simulink model "Test_Model_HR12_2016"  (R2016b)
settings: Solver=FixedStepAuto  StartTime=0.0  StopTime=length(ipoint)  FixedStep=dt  RelTol=1e-3
values from neighbouring files (symbols this model uses):
  Cbx_cyl_fill_efy_intk_mfld_prs_atm_prs_cor_cho = true    [Calib_mdl_RSA.m]
  Cbx_cyl_fill_efy_opt_cho = false    [Calib_mdl_RSA.m]
  Cbx_cyl_fill_igr_opt_cho = false    [Calib_mdl_RSA.m]
  Cbx_ex_vvt_conf = true    [Calib_mdl_RSA.m]
  Cnx_cyl_fill_ex_mfld_prs_cor_cho = 0    [Cal_basic.m]
  Cnx_cyl_nr_conf = 3    [Cal_basic.m]
  Cxx_cyl_fill_efy_drv_max = 20    [Calib_mdl_RSA.m]
  Cxx_cyl_fill_efy_dyn_max = 0.15    [Calib_mdl_RSA.m]
  Cxx_cyl_fill_efy_dyn_min = 0    [Calib_mdl_RSA.m]
  Cxx_cyl_fill_efy_dz = 0.45    [Calib_mdl_RSA.m]
  Cxx_cyl_fill_efy_ovlp_angl = 66    [Calib_mdl_RSA.m]
  Cxx_cyl_fill_efy_vvt_ofs = 0    [Calib_mdl_RSA.m]
  Cxx_cyl_fill_trap_area_h_thd = 0.2    [Cal_basic.m]
  Cxx_cyl_fill_trap_area_l_thd = 0.1    [Cal_basic.m]
  Cxx_cyl_fill_trap_efy_dz_l_thd = 1    [Cal_basic.m]
  Cxx_cyl_fill_trap_efy_dz_neg_slop = -0.5    [Cal_basic.m]
  Cxx_cyl_fill_trap_efy_dz_pos_slop = 0.5    [Cal_basic.m]
  Cxx_cyl_fill_trap_vvt_ovlp_angl = 120    [Calib_mdl_RSA.m]
  Cxx_cyl_vol = 3.9961e-04*3    (= 0.00119883)    [Cal_basic.m]    (also in Calib_mdl_RSA.m = 0.00119900004938)
  Cxx_min_cyl_fill_mdl_ex_mfld_prs_rat_cor = 0    [Cal_basic.m]
  Nnx_eng_run_stt = 2    [Calib_mdl_RSA.m]
  Nxx_atm_kpa = 101.3    [Cal_basic.m]
  Nxx_k_degc = 273.15    [Cal_basic.m]
  Nxx_kilo_bas = 1000    [Cal_basic.m]
  Nxx_wht_pgc_j_kg = 287    [Cal_basic.m]
undefined symbols (not defined in the file or in its folder): Cxx_egr_spc_heat, Cxx_thr_spc_heat, docblock, MapFilling_Aspirated
libraries: AEMS_Standard_Library x78, simulink x2
(part 1 of 5)
settings Model: Creator=a002701  LastModifiedBy=a002701

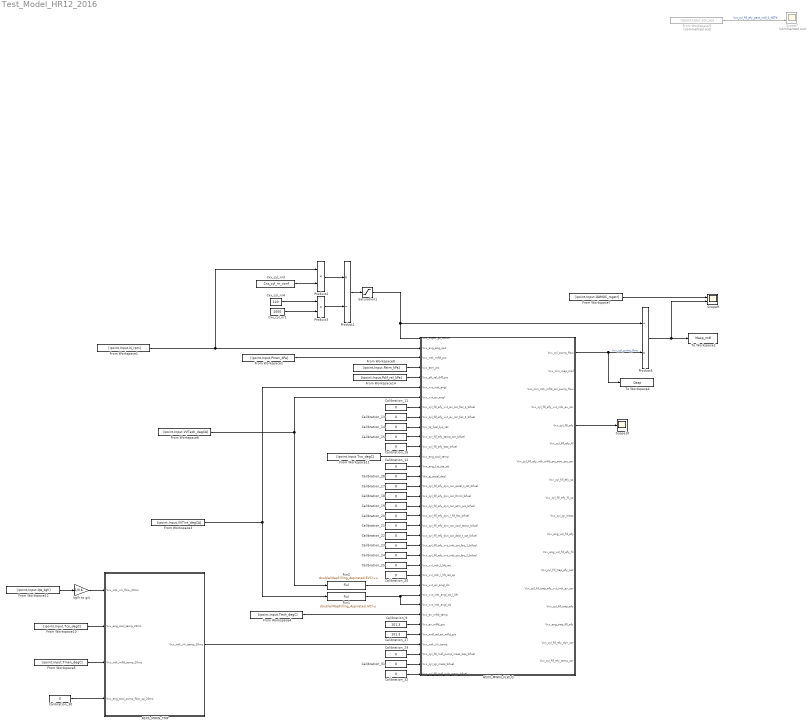
== system Test_Model_HR12_2016 ==
  ASXX_MWIN_FLW_G : Subsystem
  ASXX_MWIN_TMP : Subsystem  Tag=[MODULE]
  Calibration_{11..26,28..32} (21 alike) : Constant  Value=0  OutDataTypeStr=Inherit: Inherit via back propagation
  Calibration_27 : Constant  Value=101.3  OutDataTypeStr=Inherit: Inherit via back propagation
  Calibration_9 : Constant  Value=101.3  OutDataTypeStr=Inherit: Inherit via back propagation
  Cxx_cyl_nr1 : Constant  Value=1000  OutDataTypeStr=single
  Cxx_cyl_nr3 : Constant  Value=Cnx_cyl_nr_conf
  Cxx_cyl_nr4 : Constant  Value=120  OutDataTypeStr=single
  Fcn1 : Fcn  Expr=double(MapFilling_Aspirated.IVC)-u
  Fcn2 : Fcn  Expr=double(MapFilling_Aspirated.EVC)+u
  From Workspace1 : FromWorkspace  VariableName=[ipoint,Input.N_rpm]  SampleTime=0  Interpolate=off  OutputAfterFinalValue=Holding final value
  From Workspace10 : FromWorkspace  VariableName=[ipoint,Input.Tco_degC]  SampleTime=1  Interpolate=off  OutputAfterFinalValue=Holding final value
  From Workspace11 : FromWorkspace  VariableName=[ipoint,Input.Tco_degC]  SampleTime=1  Interpolate=off  OutputAfterFinalValue=Holding final value
  From Workspace12 : FromWorkspace  VariableName=[ipoint,Input.QA_kgh]  SampleTime=1  Interpolate=off  OutputAfterFinalValue=Holding final value
  From Workspace14 : FromWorkspace  VariableName=[ipoint,Input.Pdif_rel_kPa]  SampleTime=1  Interpolate=off  OutputAfterFinalValue=Holding final value
  From Workspace2 : FromWorkspace  VariableName=[ipoint,Input.Pman_kPa]  SampleTime=0  Interpolate=off  OutputAfterFinalValue=Holding final value
  From Workspace3 : FromWorkspace  VariableName=[ipoint,Input.VVTint_degCA]  SampleTime=0  Interpolate=off  OutputAfterFinalValue=Holding final value
  From Workspace4 : FromWorkspace  VariableName=[ipoint,Input.Texh_degC]  SampleTime=0  Interpolate=off  OutputAfterFinalValue=Holding final value
  From Workspace5 : FromWorkspace  VariableName=[ipoint,Input.Tman_degC]  SampleTime=0  Interpolate=off  OutputAfterFinalValue=Holding final value
  From Workspace6 : FromWorkspace  VariableName=[ipoint,Input.VVTexh_degCA]  SampleTime=0  Interpolate=off  OutputAfterFinalValue=Holding final value
  From Workspace7 : FromWorkspace  VariableName=[ipoint,Input.QAMGC_mgstr]  SampleTime=1  Interpolate=off  OutputAfterFinalValue=Holding final value
  From Workspace8 : FromWorkspace  VariableName=[ipoint,Input.Patm_kPa]  SampleTime=1  Interpolate=off  OutputAfterFinalValue=Holding final value
  From Workspace9 : FromWorkspace  Commented=on  VariableName=[ipoint,Input.eta_wu]  SampleTime=1  Interpolate=off  OutputAfterFinalValue=Holding final value
  Product1 : Product  Inputs=*/  OutDataTypeStr=Inherit: Inherit via back propagation
  Product2 : Product  Inputs=**  OutDataTypeStr=Inherit: Inherit via back propagation
  Product3 : Product  Inputs=**  OutDataTypeStr=Inherit: Inherit via back propagation
  Product5 : Product  Inputs=/*  OutDataTypeStr=Inherit: Inherit via back propagation
  Saturation1 : Saturate  UpperLimit=1  LowerLimit=0
      settings: AttributesFormatString=<limits=%<UpperLimit>/%<LowerLimit>>
  Scope10 : Scope
  Scope7 : Scope  Commented=on  NumInputPorts=2
  Scope9 : Scope  NumInputPorts=2
  To Workspace2 : ToWorkspace  VariableName=Masp_mdl  SampleTime=1
  To Workspace4 : ToWorkspace  VariableName=Qasp  SampleTime=1
  kg/h to g/s : Gain  Gain=1/3.6
  wires:
  From Workspace3/1 -> Fcn1/1, ASXX_MWIN_FLW_G/6(Vxx_vvt_intk_angl)
  From Workspace6/1 -> Fcn2/1, ASXX_MWIN_FLW_G/7(Vxx_vvt_ex_angl)
  ASXX_MWIN_TMP/1(Vxx_intk_vlv_temp_20ms) -> ASXX_MWIN_FLW_G/32(Vxx_intk_vlv_temp)
  From Workspace2/1 -> ASXX_MWIN_FLW_G/3(Vxx_intk_mfld_prs)
  From Workspace4/1 -> ASXX_MWIN_FLW_G/29(Vxx_ex_mfld_temp)
  Fcn1/1 -> ASXX_MWIN_FLW_G/27(Vxx_vvt_intk_angl_cls_l_lift), ASXX_MWIN_FLW_G/28(Vxx_vvt_intk_angl_cls)
  Fcn2/1 -> ASXX_MWIN_FLW_G/26(Vxx_vvt_ex_angl_cls)
  From Workspace7/1 -> Scope9/1
  Product2/1 -> Product1/1
  Product1/1 -> Saturation1/1
  Product3/1 -> Product1/2
  From Workspace1/1 -> Product2/1, ASXX_MWIN_FLW_G/2(Vxx_avg_eng_spd)
  Cxx_cyl_nr4/1 -> Product3/1
  Cxx_cyl_nr1/1 -> Product3/2
  Cxx_cyl_nr3/1 -> Product2/2
  Saturation1/1 -> ASXX_MWIN_FLW_G/1(Vxx_mgstr_gs_convs), Product5/1
  From Workspace9/1 -> Scope7/2  "Vxt_cyl_fill_efy_para_mdl_0_XETK"
  From Workspace14/1 -> ASXX_MWIN_FLW_G/5(Vxx_pft_rel_diff_prs)
  Calibration_11/1 -> ASXX_MWIN_FLW_G/8(Vxx_cyl_fill_efy_vvt_ex_cor_fac_1_bifuel)
  Calibration_13/1 -> ASXX_MWIN_FLW_G/9(Vxx_cyl_fill_efy_vvt_ex_cor_fac_2_bifuel)
  Calibration_14/1 -> ASXX_MWIN_FLW_G/10(Vxx_tq_fuel_typ_rat)
  Calibration_15/1 -> ASXX_MWIN_FLW_G/11(Vxx_cyl_fill_efy_temp_cor_bifuel)
  Calibration_16/1 -> ASXX_MWIN_FLW_G/12(Vxx_cyl_fill_efy_bas_bifuel)
  Calibration_17/1 -> ASXX_MWIN_FLW_G/16(Vxx_cyl_fill_efy_dyn_cor_accel_t_cst_bifuel)
  Calibration_18/1 -> ASXX_MWIN_FLW_G/17(Vxx_cyl_fill_efy_dyn_cor_thrml_bifuel)
  Calibration_19/1 -> ASXX_MWIN_FLW_G/18(Vxx_cyl_fill_efy_dyn_cor_atm_prs_bifuel)
  Calibration_20/1 -> ASXX_MWIN_FLW_G/19(Vxx_cyl_fill_efy_dyn_l_fill_fac_bifuel)
  Calibration_21/1 -> ASXX_MWIN_FLW_G/20(Vxx_cyl_fill_efy_dyn_cor_cool_temp_bifuel)
  Calibration_22/1 -> ASXX_MWIN_FLW_G/21(Vxx_cyl_fill_efy_dyn_cor_decl_t_cst_bifuel)
  Calibration_23/1 -> ASXX_MWIN_FLW_G/22(Vxx_cyl_fill_efy_vvt_intk_cor_fac_1_bifuel)
  Calibration_24/1 -> ASXX_MWIN_FLW_G/23(Vxx_cyl_fill_efy_vvt_intk_cor_fac_2_bifuel)
  Calibration_25/1 -> ASXX_MWIN_FLW_G/24(Vxx_vvl_intk_l_lift_rat)
  Calibration_26/1 -> ASXX_MWIN_FLW_G/25(Vxx_vvl_intk_l_lift_rat_sp)
  Calibration_27/1 -> ASXX_MWIN_FLW_G/31(Vxx_mdl_ref_ex_mfld_prs)
  Calibration_12/1 -> ASXX_MWIN_FLW_G/14(Vnx_eng_1st_sta_stt)
  Calibration_28/1 -> ASXX_MWIN_FLW_G/15(Vbx_aj_accel_decl)
  From Workspace8/1 -> ASXX_MWIN_FLW_G/4(Vxx_atm_prs)
  Calibration_9/1 -> ASXX_MWIN_FLW_G/30(Vxx_ex_mfld_prs)
  From Workspace11/1 -> ASXX_MWIN_FLW_G/13(Vxx_eng_cool_temp)
  ASXX_MWIN_FLW_G/1(Vxx_cyl_pump_flow) -> To Workspace4/1, Product5/2  "Vxx_cyl_pump_flow"
  Product5/1 -> Scope9/2, To Workspace2/1
  ASXX_MWIN_FLW_G/5(Vxx_cyl_fill_efy) -> Scope10/1
  Calibration_30/1 -> ASXX_MWIN_TMP/4(Vxx_eng_cool_pump_flow_sp_20ms)
  From Workspace10/1 -> ASXX_MWIN_TMP/2(Vxx_eng_cool_temp_20ms)
  From Workspace5/1 -> ASXX_MWIN_TMP/3(Vxx_intk_mfld_temp_20ms)
  From Workspace12/1 -> kg/h to g/s/1
  kg/h to g/s/1 -> ASXX_MWIN_TMP/1(Vxx_intk_vlv_flow_20ms)
  Calibration_29/1 -> ASXX_MWIN_FLW_G/33(Vxx_cyl_fill_mdl_pump_mass_bas_bifuel)
  Calibration_31/1 -> ASXX_MWIN_FLW_G/34(Vxx_cyl_igr_mass_bifuel)
  Calibration_32/1 -> ASXX_MWIN_FLW_G/35(Vxx_cyl_fill_mdl_ovlp_mass_bifuel)

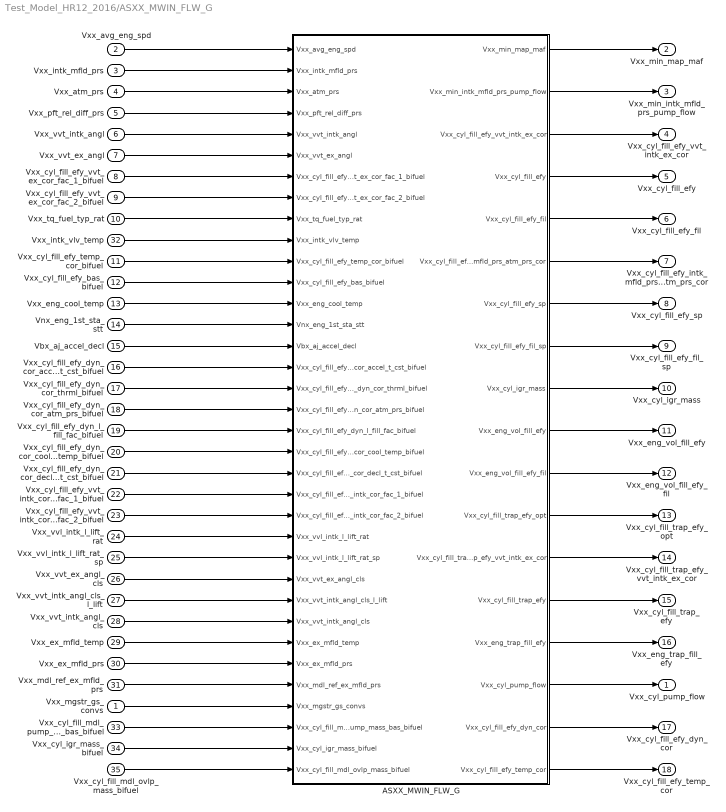
== system Test_Model_HR12_2016/ASXX_MWIN_FLW_G ==
  Vxx_mgstr_gs_convs : Inport
  Vxx_avg_eng_spd : Inport  Port=2
  Vxx_intk_mfld_prs : Inport  Port=3
  Vxx_atm_prs : Inport  Port=4
  Vxx_pft_rel_diff_prs : Inport  Port=5
  Vxx_vvt_intk_angl : Inport  Port=6
  Vxx_vvt_ex_angl : Inport  Port=7
  Vxx_cyl_fill_efy_vvt_ex_cor_fac_1_bifuel : Inport  Port=8
  Vxx_cyl_fill_efy_vvt_ex_cor_fac_2_bifuel : Inport  Port=9
  Vxx_tq_fuel_typ_rat : Inport  Port=10
  Vxx_cyl_fill_efy_temp_cor_bifuel : Inport  Port=11
  Vxx_cyl_fill_efy_bas_bifuel : Inport  Port=12
  Vxx_eng_cool_temp : Inport  Port=13
  Vnx_eng_1st_sta_stt : Inport  Port=14
  Vbx_aj_accel_decl : Inport  Port=15
  Vxx_cyl_fill_efy_dyn_cor_accel_t_cst_bifuel : Inport  Port=16
  Vxx_cyl_fill_efy_dyn_cor_thrml_bifuel : Inport  Port=17
  Vxx_cyl_fill_efy_dyn_cor_atm_prs_bifuel : Inport  Port=18
  Vxx_cyl_fill_efy_dyn_l_fill_fac_bifuel : Inport  Port=19
  Vxx_cyl_fill_efy_dyn_cor_cool_temp_bifuel : Inport  Port=20
  Vxx_cyl_fill_efy_dyn_cor_decl_t_cst_bifuel : Inport  Port=21
  Vxx_cyl_fill_efy_vvt_intk_cor_fac_1_bifuel : Inport  Port=22
  Vxx_cyl_fill_efy_vvt_intk_cor_fac_2_bifuel : Inport  Port=23
  Vxx_vvl_intk_l_lift_rat : Inport  Port=24
  Vxx_vvl_intk_l_lift_rat_sp : Inport  Port=25
  Vxx_vvt_ex_angl_cls : Inport  Port=26
  Vxx_vvt_intk_angl_cls_l_lift : Inport  Port=27
  Vxx_vvt_intk_angl_cls : Inport  Port=28
  Vxx_ex_mfld_temp : Inport  Port=29
  Vxx_ex_mfld_prs : Inport  Port=30
  Vxx_mdl_ref_ex_mfld_prs : Inport  Port=31
  Vxx_intk_vlv_temp : Inport  Port=32
  Vxx_cyl_fill_mdl_pump_mass_bas_bifuel : Inport  Port=33
  Vxx_cyl_igr_mass_bifuel : Inport  Port=34
  Vxx_cyl_fill_mdl_ovlp_mass_bifuel : Inport  Port=35
  ASXX_MWIN_FLW_G : Subsystem  Tag=[MODULE]
  Vxx_cyl_pump_flow : Outport
  Vxx_min_map_maf : Outport  Port=2
  Vxx_min_intk_mfld_prs_pump_flow : Outport  Port=3
  Vxx_cyl_fill_efy_vvt_intk_ex_cor : Outport  Port=4
  Vxx_cyl_fill_efy : Outport  Port=5
  Vxx_cyl_fill_efy_fil : Outport  Port=6
  Vxx_cyl_fill_efy_intk_mfld_prs_atm_prs_cor : Outport  Port=7
  Vxx_cyl_fill_efy_sp : Outport  Port=8
  Vxx_cyl_fill_efy_fil_sp : Outport  Port=9
  Vxx_cyl_igr_mass : Outport  Port=10
  Vxx_eng_vol_fill_efy : Outport  Port=11
  Vxx_eng_vol_fill_efy_fil : Outport  Port=12
  Vxx_cyl_fill_trap_efy_opt : Outport  Port=13
  Vxx_cyl_fill_trap_efy_vvt_intk_ex_cor : Outport  Port=14
  Vxx_cyl_fill_trap_efy : Outport  Port=15
  Vxx_eng_trap_fill_efy : Outport  Port=16
  Vxx_cyl_fill_efy_dyn_cor : Outport  Port=17
  Vxx_cyl_fill_efy_temp_cor : Outport  Port=18
  wires:
  Vbx_aj_accel_decl/1 -> ASXX_MWIN_FLW_G/15(Vbx_aj_accel_decl)
  ASXX_MWIN_FLW_G/15(Vxx_eng_trap_fill_efy) -> Vxx_eng_trap_fill_efy/1
  ASXX_MWIN_FLW_G/4(Vxx_cyl_fill_efy) -> Vxx_cyl_fill_efy/1
  ASXX_MWIN_FLW_G/11(Vxx_eng_vol_fill_efy_fil) -> Vxx_eng_vol_fill_efy_fil/1
  Vxx_cyl_fill_efy_dyn_cor_cool_temp_bifuel/1 -> ASXX_MWIN_FLW_G/20(Vxx_cyl_fill_efy_dyn_cor_cool_temp_bifuel)
  Vnx_eng_1st_sta_stt/1 -> ASXX_MWIN_FLW_G/14(Vnx_eng_1st_sta_stt)
  Vxx_cyl_fill_efy_dyn_cor_accel_t_cst_bifuel/1 -> ASXX_MWIN_FLW_G/16(Vxx_cyl_fill_efy_dyn_cor_accel_t_cst_bifuel)
  ASXX_MWIN_FLW_G/14(Vxx_cyl_fill_trap_efy) -> Vxx_cyl_fill_trap_efy/1
  ASXX_MWIN_FLW_G/9(Vxx_cyl_igr_mass) -> Vxx_cyl_igr_mass/1
  ASXX_MWIN_FLW_G/12(Vxx_cyl_fill_trap_efy_opt) -> Vxx_cyl_fill_trap_efy_opt/1
  ASXX_MWIN_FLW_G/13(Vxx_cyl_fill_trap_efy_vvt_intk_ex_cor) -> Vxx_cyl_fill_trap_efy_vvt_intk_ex_cor/1
  Vxx_cyl_fill_efy_dyn_l_fill_fac_bifuel/1 -> ASXX_MWIN_FLW_G/19(Vxx_cyl_fill_efy_dyn_l_fill_fac_bifuel)
  Vxx_cyl_fill_efy_dyn_cor_atm_prs_bifuel/1 -> ASXX_MWIN_FLW_G/18(Vxx_cyl_fill_efy_dyn_cor_atm_prs_bifuel)
  Vxx_ex_mfld_temp/1 -> ASXX_MWIN_FLW_G/29(Vxx_ex_mfld_temp)
  Vxx_cyl_fill_efy_bas_bifuel/1 -> ASXX_MWIN_FLW_G/12(Vxx_cyl_fill_efy_bas_bifuel)
  ASXX_MWIN_FLW_G/2(Vxx_min_intk_mfld_prs_pump_flow) -> Vxx_min_intk_mfld_prs_pump_flow/1
  ASXX_MWIN_FLW_G/6(Vxx_cyl_fill_efy_intk_mfld_prs_atm_prs_cor) -> Vxx_cyl_fill_efy_intk_mfld_prs_atm_prs_cor/1
  Vxx_cyl_fill_efy_temp_cor_bifuel/1 -> ASXX_MWIN_FLW_G/11(Vxx_cyl_fill_efy_temp_cor_bifuel)
  ASXX_MWIN_FLW_G/8(Vxx_cyl_fill_efy_fil_sp) -> Vxx_cyl_fill_efy_fil_sp/1
  ASXX_MWIN_FLW_G/16(Vxx_cyl_pump_flow) -> Vxx_cyl_pump_flow/1
  ASXX_MWIN_FLW_G/5(Vxx_cyl_fill_efy_fil) -> Vxx_cyl_fill_efy_fil/1
  ASXX_MWIN_FLW_G/7(Vxx_cyl_fill_efy_sp) -> Vxx_cyl_fill_efy_sp/1
  ASXX_MWIN_FLW_G/1(Vxx_min_map_maf) -> Vxx_min_map_maf/1
  ASXX_MWIN_FLW_G/3(Vxx_cyl_fill_efy_vvt_intk_ex_cor) -> Vxx_cyl_fill_efy_vvt_intk_ex_cor/1
  Vxx_vvt_intk_angl/1 -> ASXX_MWIN_FLW_G/5(Vxx_vvt_intk_angl)
  Vxx_cyl_fill_efy_vvt_ex_cor_fac_2_bifuel/1 -> ASXX_MWIN_FLW_G/8(Vxx_cyl_fill_efy_vvt_ex_cor_fac_2_bifuel)
  Vxx_avg_eng_spd/1 -> ASXX_MWIN_FLW_G/1(Vxx_avg_eng_spd)
  Vxx_intk_mfld_prs/1 -> ASXX_MWIN_FLW_G/2(Vxx_intk_mfld_prs)
  Vxx_cyl_fill_efy_vvt_intk_cor_fac_1_bifuel/1 -> ASXX_MWIN_FLW_G/22(Vxx_cyl_fill_efy_vvt_intk_cor_fac_1_bifuel)
  Vxx_cyl_fill_efy_dyn_cor_thrml_bifuel/1 -> ASXX_MWIN_FLW_G/17(Vxx_cyl_fill_efy_dyn_cor_thrml_bifuel)
  Vxx_atm_prs/1 -> ASXX_MWIN_FLW_G/3(Vxx_atm_prs)
  Vxx_pft_rel_diff_prs/1 -> ASXX_MWIN_FLW_G/4(Vxx_pft_rel_diff_prs)
  Vxx_vvt_ex_angl/1 -> ASXX_MWIN_FLW_G/6(Vxx_vvt_ex_angl)
  Vxx_tq_fuel_typ_rat/1 -> ASXX_MWIN_FLW_G/9(Vxx_tq_fuel_typ_rat)
  Vxx_vvl_intk_l_lift_rat/1 -> ASXX_MWIN_FLW_G/24(Vxx_vvl_intk_l_lift_rat)
  Vxx_vvl_intk_l_lift_rat_sp/1 -> ASXX_MWIN_FLW_G/25(Vxx_vvl_intk_l_lift_rat_sp)
  Vxx_vvt_ex_angl_cls/1 -> ASXX_MWIN_FLW_G/26(Vxx_vvt_ex_angl_cls)
  Vxx_vvt_intk_angl_cls/1 -> ASXX_MWIN_FLW_G/28(Vxx_vvt_intk_angl_cls)
  Vxx_ex_mfld_prs/1 -> ASXX_MWIN_FLW_G/30(Vxx_ex_mfld_prs)
  Vxx_vvt_intk_angl_cls_l_lift/1 -> ASXX_MWIN_FLW_G/27(Vxx_vvt_intk_angl_cls_l_lift)
  ASXX_MWIN_FLW_G/10(Vxx_eng_vol_fill_efy) -> Vxx_eng_vol_fill_efy/1
  Vxx_mdl_ref_ex_mfld_prs/1 -> ASXX_MWIN_FLW_G/31(Vxx_mdl_ref_ex_mfld_prs)
  Vxx_cyl_fill_efy_dyn_cor_decl_t_cst_bifuel/1 -> ASXX_MWIN_FLW_G/21(Vxx_cyl_fill_efy_dyn_cor_decl_t_cst_bifuel)
  Vxx_cyl_fill_efy_vvt_ex_cor_fac_1_bifuel/1 -> ASXX_MWIN_FLW_G/7(Vxx_cyl_fill_efy_vvt_ex_cor_fac_1_bifuel)
  Vxx_cyl_fill_efy_vvt_intk_cor_fac_2_bifuel/1 -> ASXX_MWIN_FLW_G/23(Vxx_cyl_fill_efy_vvt_intk_cor_fac_2_bifuel)
  Vxx_mgstr_gs_convs/1 -> ASXX_MWIN_FLW_G/32(Vxx_mgstr_gs_convs)
  Vxx_eng_cool_temp/1 -> ASXX_MWIN_FLW_G/13(Vxx_eng_cool_temp)
  Vxx_intk_vlv_temp/1 -> ASXX_MWIN_FLW_G/10(Vxx_intk_vlv_temp)
  ASXX_MWIN_FLW_G/17(Vxx_cyl_fill_efy_dyn_cor) -> Vxx_cyl_fill_efy_dyn_cor/1
  ASXX_MWIN_FLW_G/18(Vxx_cyl_fill_efy_temp_cor) -> Vxx_cyl_fill_efy_temp_cor/1
  Vxx_cyl_fill_mdl_pump_mass_bas_bifuel/1 -> ASXX_MWIN_FLW_G/33(Vxx_cyl_fill_mdl_pump_mass_bas_bifuel)
  Vxx_cyl_igr_mass_bifuel/1 -> ASXX_MWIN_FLW_G/34(Vxx_cyl_igr_mass_bifuel)
  Vxx_cyl_fill_mdl_ovlp_mass_bifuel/1 -> ASXX_MWIN_FLW_G/35(Vxx_cyl_fill_mdl_ovlp_mass_bifuel)

== system Test_Model_HR12_2016/ASXX_MWIN_TMP ==
  Vxx_intk_vlv_flow_20ms : Inport  Interpolate=off
  Vxx_eng_cool_temp_20ms : Inport  Port=2  Interpolate=off
  Vxx_intk_mfld_temp_20ms : Inport  Port=3  Interpolate=off
  Vxx_eng_cool_pump_flow_sp_20ms : Inport  Port=4  Interpolate=off
  ASXX_MWIN_TMP_ivlvtmd_20ms : Subsystem  Tag=[RUNNABLE]  TreatAsAtomicUnit=on
      settings: AttributesFormatString=%<TAG>
  Manual Switch : ManualSwitch
  Vxx_intk_vlv_temp_20ms : Outport
  wires:
  Manual Switch/1 -> Vxx_intk_vlv_temp_20ms/1
  Vxx_eng_cool_temp_20ms/1 -> ASXX_MWIN_TMP_ivlvtmd_20ms/2(Vxx_eng_cool_temp_20ms)
  Vxx_intk_mfld_temp_20ms/1 -> Manual Switch/2, ASXX_MWIN_TMP_ivlvtmd_20ms/3(Vxx_intk_mfld_temp_20ms)
  Vxx_intk_vlv_flow_20ms/1 -> ASXX_MWIN_TMP_ivlvtmd_20ms/1(Vxx_intk_vlv_flow_20ms)
  Vxx_eng_cool_pump_flow_sp_20ms/1 -> ASXX_MWIN_TMP_ivlvtmd_20ms/4(Vxx_eng_cool_pump_flow_sp_20ms)
  ASXX_MWIN_TMP_ivlvtmd_20ms/1(Vxx_intk_vlv_temp_20ms) -> Manual Switch/1

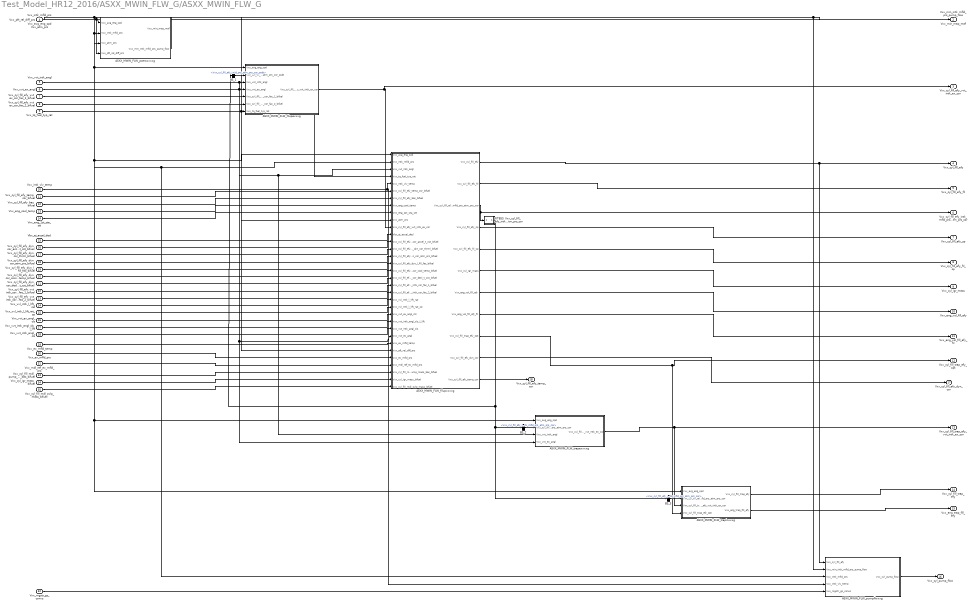
== system Test_Model_HR12_2016/ASXX_MWIN_FLW_G/ASXX_MWIN_FLW_G ==
  Vxx_avg_eng_spd : Inport
  Vxx_intk_mfld_prs : Inport  Port=2
  Vxx_atm_prs : Inport  Port=3
  Vxx_pft_rel_diff_prs : Inport  Port=4
  Vxx_vvt_intk_angl : Inport  Port=5
  Vxx_vvt_ex_angl : Inport  Port=6
  Vxx_cyl_fill_efy_vvt_ex_cor_fac_1_bifuel : Inport  Port=7
  Vxx_cyl_fill_efy_vvt_ex_cor_fac_2_bifuel : Inport  Port=8
  Vxx_tq_fuel_typ_rat : Inport  Port=9
  Vxx_intk_vlv_temp : Inport  Port=10
  Vxx_cyl_fill_efy_temp_cor_bifuel : Inport  Port=11
  Vxx_cyl_fill_efy_bas_bifuel : Inport  Port=12
  Vxx_eng_cool_temp : Inport  Port=13
  Vnx_eng_1st_sta_stt : Inport  Port=14
  Vbx_aj_accel_decl : Inport  Port=15
  Vxx_cyl_fill_efy_dyn_cor_accel_t_cst_bifuel : Inport  Port=16
  Vxx_cyl_fill_efy_dyn_cor_thrml_bifuel : Inport  Port=17
  Vxx_cyl_fill_efy_dyn_cor_atm_prs_bifuel : Inport  Port=18
  Vxx_cyl_fill_efy_dyn_l_fill_fac_bifuel : Inport  Port=19
  Vxx_cyl_fill_efy_dyn_cor_cool_temp_bifuel : Inport  Port=20
  Vxx_cyl_fill_efy_dyn_cor_decl_t_cst_bifuel : Inport  Port=21
  Vxx_cyl_fill_efy_vvt_intk_cor_fac_1_bifuel : Inport  Port=22
  Vxx_cyl_fill_efy_vvt_intk_cor_fac_2_bifuel : Inport  Port=23
  Vxx_vvl_intk_l_lift_rat : Inport  Port=24
  Vxx_vvl_intk_l_lift_rat_sp : Inport  Port=25
  Vxx_vvt_ex_angl_cls : Inport  Port=26
  Vxx_vvt_intk_angl_cls_l_lift : Inport  Port=27
  Vxx_vvt_intk_angl_cls : Inport  Port=28
  Vxx_ex_mfld_temp : Inport  Port=29
  Vxx_ex_mfld_prs : Inport  Port=30
  Vxx_mdl_ref_ex_mfld_prs : Inport  Port=31
  Vxx_mgstr_gs_convs : Inport  Port=32
  Vxx_cyl_fill_mdl_pump_mass_bas_bifuel : Inport  Port=33
  Vxx_cyl_igr_mass_bifuel : Inport  Port=34
  Vxx_cyl_fill_mdl_ovlp_mass_bifuel : Inport  Port=35
  ASXX_MWIN_FLW_filupexxxg : Subsystem
  ASXX_MWIN_FLW_filupxxxxg : Subsystem
  ASXX_MWIN_FLW_pumpflwxxg : Subsystem
  ASXX_MWIN_FLW_pzeroxxxxg : Subsystem
  ASXX_MWIN_FLW_trapexxxxg : Subsystem
  ASXX_MWIN_FLW_trapinxxxg : Subsystem
  BS_1 : BusSelector  OutputSignals=Vxx_cyl_fill_efy_intk_mfld_prs_atm_prs_cor_pudt
  BS_2 : BusSelector  OutputSignals=Vxx_cyl_fill_efy_intk_mfld_prs_atm_prs_cor
  BS_3 : BusSelector  OutputSignals=Vxx_cyl_fill_efy_intk_mfld_prs_atm_prs_cor
  RTBSS_Vxx_cyl_fill_efy_intk_mfld_prs_atm_prs_cor : Subsystem
  Vxx_min_map_maf : Outport
  Vxx_min_intk_mfld_prs_pump_flow : Outport  Port=2
  Vxx_cyl_fill_efy_vvt_intk_ex_cor : Outport  Port=3
  Vxx_cyl_fill_efy : Outport  Port=4
  Vxx_cyl_fill_efy_fil : Outport  Port=5
  Vxx_cyl_fill_efy_intk_mfld_prs_atm_prs_cor : Outport  Port=6
  Vxx_cyl_fill_efy_sp : Outport  Port=7
  Vxx_cyl_fill_efy_fil_sp : Outport  Port=8
  Vxx_cyl_igr_mass : Outport  Port=9
  Vxx_eng_vol_fill_efy : Outport  Port=10
  Vxx_eng_vol_fill_efy_fil : Outport  Port=11
  Vxx_cyl_fill_trap_efy_opt : Outport  Port=12
  Vxx_cyl_fill_trap_efy_vvt_intk_ex_cor : Outport  Port=13
  Vxx_cyl_fill_trap_efy : Outport  Port=14
  Vxx_eng_trap_fill_efy : Outport  Port=15
  Vxx_cyl_pump_flow : Outport  Port=16
  Vxx_cyl_fill_efy_dyn_cor : Outport  Port=17
  Vxx_cyl_fill_efy_temp_cor : Outport  Port=18
  wires:
  Vxx_intk_vlv_temp/1 -> ASXX_MWIN_FLW_pumpflwxxg/4(Vxx_intk_vlv_temp), ASXX_MWIN_FLW_filupxxxxg/5(Vxx_intk_vlv_temp)
  Vxx_tq_fuel_typ_rat/1 -> ASXX_MWIN_FLW_filupxxxxg/4(Vxx_tq_fuel_typ_rat), ASXX_MWIN_FLW_filupexxxg/7(Vxx_tq_fuel_typ_rat)
  Vxx_vvt_ex_angl/1 -> ASXX_MWIN_FLW_filupexxxg/4(Vxx_vvt_ex_angl), ASXX_MWIN_FLW_trapexxxxg/4(Vxx_vvt_ex_angl), ASXX_MWIN_FLW_filupxxxxg/26(Vxx_vvt_ex_angl)
  Vxx_vvt_intk_angl/1 -> ASXX_MWIN_FLW_filupexxxg/3(Vxx_vvt_intk_angl), ASXX_MWIN_FLW_trapexxxxg/3(Vxx_vvt_intk_angl), ASXX_MWIN_FLW_filupxxxxg/3(Vxx_vvt_intk_angl)
  Vxx_pft_rel_diff_prs/1 -> ASXX_MWIN_FLW_filupxxxxg/28(Vxx_pft_rel_diff_prs), ASXX_MWIN_FLW_pzeroxxxxg/4(Vxx_pft_rel_diff_prs)
  Vxx_atm_prs/1 -> ASXX_MWIN_FLW_filupxxxxg/10(Vxx_atm_prs), ASXX_MWIN_FLW_pzeroxxxxg/3(Vxx_atm_prs)
  Vxx_intk_mfld_prs/1 -> ASXX_MWIN_FLW_pzeroxxxxg/2(Vxx_intk_mfld_prs), ASXX_MWIN_FLW_pumpflwxxg/3(Vxx_intk_mfld_prs), ASXX_MWIN_FLW_filupxxxxg/2(Vxx_intk_mfld_prs)
  Vxx_avg_eng_spd/1 -> ASXX_MWIN_FLW_filupexxxg/1(Vxx_avg_eng_spd), ASXX_MWIN_FLW_filupxxxxg/1(Vxx_avg_eng_spd), ASXX_MWIN_FLW_trapinxxxg/1(Vxx_avg_eng_spd), ASXX_MWIN_FLW_trapexxxxg/1(Vxx_avg_eng_spd), ASXX_MWIN_FLW_pzeroxxxxg/1(Vxx_avg_eng_spd)
  RTBSS_Vxx_cyl_fill_efy_intk_mfld_prs_atm_prs_cor/1(Vxx_cyl_fill_efy_intk_mfld_prs_atm_prs_cor_rt) -> BS_3/1, BS_2/1, BS_1/1
  BS_1/1 -> ASXX_MWIN_FLW_filupexxxg/2(Vxx_cyl_fill_efy_intk_mfld_prs_atm_prs_cor_pudt)  "<Vxx_cyl_fill_efy_intk_mfld_prs_atm_prs_cor_pudt>"
  Vxx_cyl_fill_efy_vvt_ex_cor_fac_1_bifuel/1 -> ASXX_MWIN_FLW_filupexxxg/5(Vxx_cyl_fill_efy_vvt_ex_cor_fac_1_bifuel)
  Vxx_cyl_fill_efy_vvt_ex_cor_fac_2_bifuel/1 -> ASXX_MWIN_FLW_filupexxxg/6(Vxx_cyl_fill_efy_vvt_ex_cor_fac_2_bifuel)
  ASXX_MWIN_FLW_filupexxxg/1(Vxx_cyl_fill_efy_vvt_intk_ex_cor) -> Vxx_cyl_fill_efy_vvt_intk_ex_cor/1, ASXX_MWIN_FLW_filupxxxxg/11(Vxx_cyl_fill_efy_vvt_intk_ex_cor)
  Vxx_cyl_fill_efy_temp_cor_bifuel/1 -> ASXX_MWIN_FLW_filupxxxxg/6(Vxx_cyl_fill_efy_temp_cor_bifuel)
  Vxx_cyl_fill_efy_bas_bifuel/1 -> ASXX_MWIN_FLW_filupxxxxg/7(Vxx_cyl_fill_efy_bas_bifuel)
  Vxx_eng_cool_temp/1 -> ASXX_MWIN_FLW_filupxxxxg/8(Vxx_eng_cool_temp)
  Vnx_eng_1st_sta_stt/1 -> ASXX_MWIN_FLW_filupxxxxg/9(Vnx_eng_1st_sta_stt)
  Vbx_aj_accel_decl/1 -> ASXX_MWIN_FLW_filupxxxxg/12(Vbx_aj_accel_decl)
  Vxx_cyl_fill_efy_dyn_cor_accel_t_cst_bifuel/1 -> ASXX_MWIN_FLW_filupxxxxg/13(Vxx_cyl_fill_efy_dyn_cor_accel_t_cst_bifuel)
  Vxx_cyl_fill_efy_dyn_cor_thrml_bifuel/1 -> ASXX_MWIN_FLW_filupxxxxg/14(Vxx_cyl_fill_efy_dyn_cor_thrml_bifuel)
  Vxx_cyl_fill_efy_dyn_cor_atm_prs_bifuel/1 -> ASXX_MWIN_FLW_filupxxxxg/15(Vxx_cyl_fill_efy_dyn_cor_atm_prs_bifuel)
  Vxx_cyl_fill_efy_dyn_l_fill_fac_bifuel/1 -> ASXX_MWIN_FLW_filupxxxxg/16(Vxx_cyl_fill_efy_dyn_l_fill_fac_bifuel)
  Vxx_cyl_fill_efy_dyn_cor_cool_temp_bifuel/1 -> ASXX_MWIN_FLW_filupxxxxg/17(Vxx_cyl_fill_efy_dyn_cor_cool_temp_bifuel)
  Vxx_cyl_fill_efy_dyn_cor_decl_t_cst_bifuel/1 -> ASXX_MWIN_FLW_filupxxxxg/18(Vxx_cyl_fill_efy_dyn_cor_decl_t_cst_bifuel)
  Vxx_cyl_fill_efy_vvt_intk_cor_fac_1_bifuel/1 -> ASXX_MWIN_FLW_filupxxxxg/19(Vxx_cyl_fill_efy_vvt_intk_cor_fac_1_bifuel)
  Vxx_cyl_fill_efy_vvt_intk_cor_fac_2_bifuel/1 -> ASXX_MWIN_FLW_filupxxxxg/20(Vxx_cyl_fill_efy_vvt_intk_cor_fac_2_bifuel)
  Vxx_vvl_intk_l_lift_rat/1 -> ASXX_MWIN_FLW_filupxxxxg/21(Vxx_vvl_intk_l_lift_rat)
  Vxx_vvl_intk_l_lift_rat_sp/1 -> ASXX_MWIN_FLW_filupxxxxg/22(Vxx_vvl_intk_l_lift_rat_sp)
  Vxx_vvt_ex_angl_cls/1 -> ASXX_MWIN_FLW_filupxxxxg/23(Vxx_vvt_ex_angl_cls)
  Vxx_vvt_intk_angl_cls_l_lift/1 -> ASXX_MWIN_FLW_filupxxxxg/24(Vxx_vvt_intk_angl_cls_l_lift)
  Vxx_vvt_intk_angl_cls/1 -> ASXX_MWIN_FLW_filupxxxxg/25(Vxx_vvt_intk_angl_cls)
  Vxx_ex_mfld_temp/1 -> ASXX_MWIN_FLW_filupxxxxg/27(Vxx_ex_mfld_temp)
  Vxx_ex_mfld_prs/1 -> ASXX_MWIN_FLW_filupxxxxg/29(Vxx_ex_mfld_prs)
  Vxx_mdl_ref_ex_mfld_prs/1 -> ASXX_MWIN_FLW_filupxxxxg/30(Vxx_mdl_ref_ex_mfld_prs)
  ASXX_MWIN_FLW_filupxxxxg/1(Vxx_cyl_fill_efy) -> ASXX_MWIN_FLW_pumpflwxxg/1(Vxx_cyl_fill_efy), Vxx_cyl_fill_efy/1
  ASXX_MWIN_FLW_filupxxxxg/2(Vxx_cyl_fill_efy_fil) -> Vxx_cyl_fill_efy_fil/1
  ASXX_MWIN_FLW_filupxxxxg/3(Vxx_cyl_fill_efy_intk_mfld_prs_atm_prs_cor) -> Vxx_cyl_fill_efy_intk_mfld_prs_atm_prs_cor/1, RTBSS_Vxx_cyl_fill_efy_intk_mfld_prs_atm_prs_cor/1(Vxx_cyl_fill_efy_intk_mfld_prs_atm_prs_cor)
  ASXX_MWIN_FLW_filupxxxxg/4(Vxx_cyl_fill_efy_sp) -> Vxx_cyl_fill_efy_sp/1
  ASXX_MWIN_FLW_filupxxxxg/5(Vxx_cyl_fill_efy_fil_sp) -> Vxx_cyl_fill_efy_fil_sp/1
  ASXX_MWIN_FLW_filupxxxxg/6(Vxx_cyl_igr_mass) -> Vxx_cyl_igr_mass/1
  ASXX_MWIN_FLW_filupxxxxg/7(Vxx_eng_vol_fill_efy) -> Vxx_eng_vol_fill_efy/1
  ASXX_MWIN_FLW_filupxxxxg/8(Vxx_eng_vol_fill_efy_fil) -> Vxx_eng_vol_fill_efy_fil/1
  ASXX_MWIN_FLW_filupxxxxg/9(Vxx_cyl_fill_trap_efy_opt) -> Vxx_cyl_fill_trap_efy_opt/1, ASXX_MWIN_FLW_trapinxxxg/4(Vxx_cyl_fill_trap_efy_opt)
  Vxx_mgstr_gs_convs/1 -> ASXX_MWIN_FLW_pumpflwxxg/5(Vxx_mgstr_gs_convs)
  ASXX_MWIN_FLW_pumpflwxxg/1(Vxx_cyl_pump_flow) -> Vxx_cyl_pump_flow/1
  ASXX_MWIN_FLW_pzeroxxxxg/1(Vxx_min_map_maf) -> Vxx_min_map_maf/1
  ASXX_MWIN_FLW_pzeroxxxxg/2(Vxx_min_intk_mfld_prs_pump_flow) -> Vxx_min_intk_mfld_prs_pump_flow/1, ASXX_MWIN_FLW_pumpflwxxg/2(Vxx_min_intk_mfld_prs_pump_flow)
  BS_2/1 -> ASXX_MWIN_FLW_trapexxxxg/2(Vxx_cyl_fill_efy_intk_mfld_prs_atm_prs_cor)  "<Vxx_cyl_fill_efy_intk_mfld_prs_atm_prs_cor>"
  ASXX_MWIN_FLW_trapexxxxg/1(Vxx_cyl_fill_trap_efy_vvt_intk_ex_cor) -> ASXX_MWIN_FLW_trapinxxxg/3(Vxx_cyl_fill_trap_efy_vvt_intk_ex_cor), Vxx_cyl_fill_trap_efy_vvt_intk_ex_cor/1
  BS_3/1 -> ASXX_MWIN_FLW_trapinxxxg/2(Vxx_cyl_fill_efy_intk_mfld_prs_atm_prs_cor)  "<Vxx_cyl_fill_efy_intk_mfld_prs_atm_prs_cor>"
  ASXX_MWIN_FLW_trapinxxxg/1(Vxx_cyl_fill_trap_efy) -> Vxx_cyl_fill_trap_efy/1
  ASXX_MWIN_FLW_trapinxxxg/2(Vxx_eng_trap_fill_efy) -> Vxx_eng_trap_fill_efy/1
  ASXX_MWIN_FLW_filupxxxxg/10(Vxx_cyl_fill_efy_dyn_cor) -> Vxx_cyl_fill_efy_dyn_cor/1
  ASXX_MWIN_FLW_filupxxxxg/11(Vxx_cyl_fill_efy_temp_cor) -> Vxx_cyl_fill_efy_temp_cor/1
  Vxx_cyl_fill_mdl_pump_mass_bas_bifuel/1 -> ASXX_MWIN_FLW_filupxxxxg/31(Vxx_cyl_fill_mdl_pump_mass_bas_bifuel)
  Vxx_cyl_igr_mass_bifuel/1 -> ASXX_MWIN_FLW_filupxxxxg/32(Vxx_cyl_igr_mass_bifuel)
  Vxx_cyl_fill_mdl_ovlp_mass_bifuel/1 -> ASXX_MWIN_FLW_filupxxxxg/33(Vxx_cyl_fill_mdl_ovlp_mass_bifuel)

== system Test_Model_HR12_2016/ASXX_MWIN_TMP/ASXX_MWIN_TMP_ivlvtmd_20ms ==
  Vxx_intk_vlv_flow_20ms : Inport  Interpolate=off
  Vxx_eng_cool_temp_20ms : Inport  Port=2  Interpolate=off
  Vxx_intk_mfld_temp_20ms : Inport  Port=3  Interpolate=off
  Vxx_eng_cool_pump_flow_sp_20ms : Inport  Port=4  Interpolate=off
  B1_INTK_VLV_MIX_TEMP : Subsystem  Commented=on
  B2_INTK_VLV_TEMP : Subsystem
  Vxx_intk_vlv_temp_20ms : Outport  InitialOutput=20
      settings: AttributesFormatString=<initial=%<InitialOutput>>\n<whendisabled=%<OutputWhenDisabled>>
  wires:
  Vxx_intk_vlv_flow_20ms/1 -> B2_INTK_VLV_TEMP/4(Vxx_intk_vlv_flow_20ms)  "Vxx_intk_vlv_flow_20ms"
  Vxx_eng_cool_temp_20ms/1 -> B2_INTK_VLV_TEMP/2(Vxx_eng_cool_temp_20ms)  "Vxx_eng_cool_temp_20ms"
  Vxx_intk_mfld_temp_20ms/1 -> B2_INTK_VLV_TEMP/1(Vxx_intk_vlv_mix_temp_20ms)
  B2_INTK_VLV_TEMP/1(Vxx_intk_vlv_temp_20ms) -> Vxx_intk_vlv_temp_20ms/1
  Vxx_eng_cool_pump_flow_sp_20ms/1 -> B2_INTK_VLV_TEMP/3(Vxx_eng_cool_pump_flow_sp_20ms)

== system Test_Model_HR12_2016/ASXX_MWIN_FLW_G/ASXX_MWIN_FLW_G/ASXX_MWIN_FLW_filupexxxg ==
  Vxx_avg_eng_spd : Inport  Interpolate=off
  Vxx_cyl_fill_efy_intk_mfld_prs_atm_prs_cor_pudt : Inport  Port=2  Interpolate=off
  Vxx_vvt_intk_angl : Inport  Port=3  Interpolate=off
  Vxx_vvt_ex_angl : Inport  Port=4  Interpolate=off
  Vxx_cyl_fill_efy_vvt_ex_cor_fac_1_bifuel : Inport  Port=5  Interpolate=off
  Vxx_cyl_fill_efy_vvt_ex_cor_fac_2_bifuel : Inport  Port=6  Interpolate=off
  Vxx_tq_fuel_typ_rat : Inport  Port=7  Interpolate=off
  ASXX_MWIN_FLW_filupexxxg_10ms : Subsystem  Tag=[RUNNABLE]  TreatAsAtomicUnit=on  RTWFileName=InAsiIaf_Filupex_xxxxxg
      settings: AttributesFormatString=%<Tag>  RTWSystemCode=Nonreusable function  RTWFcnNameOpts=Use subsystem name  RTWFileNameOpts=User specified
  Vxx_cyl_fill_efy_vvt_intk_ex_cor : Outport
  wires:
  Vxx_cyl_fill_efy_intk_mfld_prs_atm_prs_cor_pudt/1 -> ASXX_MWIN_FLW_filupexxxg_10ms/2(Vxx_cyl_fill_efy_intk_mfld_prs_atm_prs_cor_pudt)
  ASXX_MWIN_FLW_filupexxxg_10ms/1(Vxx_cyl_fill_efy_vvt_intk_ex_cor) -> Vxx_cyl_fill_efy_vvt_intk_ex_cor/1
  Vxx_tq_fuel_typ_rat/1 -> ASXX_MWIN_FLW_filupexxxg_10ms/7(Vxx_tq_fuel_typ_rat)
  Vxx_vvt_ex_angl/1 -> ASXX_MWIN_FLW_filupexxxg_10ms/4(Vxx_vvt_ex_angl)
  Vxx_vvt_intk_angl/1 -> ASXX_MWIN_FLW_filupexxxg_10ms/3(Vxx_vvt_intk_angl)
  Vxx_avg_eng_spd/1 -> ASXX_MWIN_FLW_filupexxxg_10ms/1(Vxx_avg_eng_spd)
  Vxx_cyl_fill_efy_vvt_ex_cor_fac_1_bifuel/1 -> ASXX_MWIN_FLW_filupexxxg_10ms/5(Vxx_cyl_fill_efy_vvt_ex_cor_fac_1_bifuel)
  Vxx_cyl_fill_efy_vvt_ex_cor_fac_2_bifuel/1 -> ASXX_MWIN_FLW_filupexxxg_10ms/6(Vxx_cyl_fill_efy_vvt_ex_cor_fac_2_bifuel)

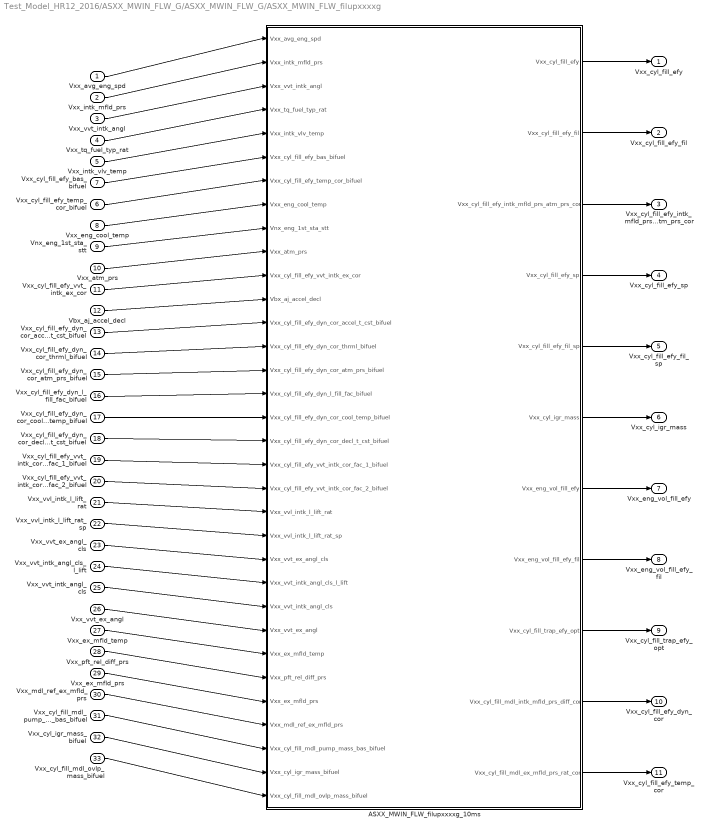
== system Test_Model_HR12_2016/ASXX_MWIN_FLW_G/ASXX_MWIN_FLW_G/ASXX_MWIN_FLW_filupxxxxg ==
  Vxx_avg_eng_spd : Inport  Interpolate=off
  Vxx_intk_mfld_prs : Inport  Port=2  Interpolate=off
  Vxx_vvt_intk_angl : Inport  Port=3  Interpolate=off
  Vxx_tq_fuel_typ_rat : Inport  Port=4  Interpolate=off
  Vxx_intk_vlv_temp : Inport  Port=5  Interpolate=off
  Vxx_cyl_fill_efy_temp_cor_bifuel : Inport  Port=6  Interpolate=off
  Vxx_cyl_fill_efy_bas_bifuel : Inport  Port=7  Interpolate=off
  Vxx_eng_cool_temp : Inport  Port=8  Interpolate=off
  Vnx_eng_1st_sta_stt : Inport  Port=9  Interpolate=off
  Vxx_atm_prs : Inport  Port=10  Interpolate=off
  Vxx_cyl_fill_efy_vvt_intk_ex_cor : Inport  Port=11  Interpolate=off
  Vbx_aj_accel_decl : Inport  Port=12  Interpolate=off
  Vxx_cyl_fill_efy_dyn_cor_accel_t_cst_bifuel : Inport  Port=13  Interpolate=off
  Vxx_cyl_fill_efy_dyn_cor_thrml_bifuel : Inport  Port=14  Interpolate=off
  Vxx_cyl_fill_efy_dyn_cor_atm_prs_bifuel : Inport  Port=15  Interpolate=off
  Vxx_cyl_fill_efy_dyn_l_fill_fac_bifuel : Inport  Port=16  Interpolate=off
  Vxx_cyl_fill_efy_dyn_cor_cool_temp_bifuel : Inport  Port=17  Interpolate=off
  Vxx_cyl_fill_efy_dyn_cor_decl_t_cst_bifuel : Inport  Port=18  Interpolate=off
  Vxx_cyl_fill_efy_vvt_intk_cor_fac_1_bifuel : Inport  Port=19  Interpolate=off
  Vxx_cyl_fill_efy_vvt_intk_cor_fac_2_bifuel : Inport  Port=20  Interpolate=off
  Vxx_vvl_intk_l_lift_rat : Inport  Port=21  Interpolate=off
  Vxx_vvl_intk_l_lift_rat_sp : Inport  Port=22  Interpolate=off
  Vxx_vvt_ex_angl_cls : Inport  Port=23  Interpolate=off
  Vxx_vvt_intk_angl_cls_l_lift : Inport  Port=24  Interpolate=off
  Vxx_vvt_intk_angl_cls : Inport  Port=25  Interpolate=off
  Vxx_vvt_ex_angl : Inport  Port=26  Interpolate=off
  Vxx_ex_mfld_temp : Inport  Port=27  Interpolate=off
  Vxx_pft_rel_diff_prs : Inport  Port=28  Interpolate=off
  Vxx_ex_mfld_prs : Inport  Port=29  Interpolate=off
  Vxx_mdl_ref_ex_mfld_prs : Inport  Port=30  Interpolate=off
  Vxx_cyl_fill_mdl_pump_mass_bas_bifuel : Inport  Port=31  Interpolate=off
  Vxx_cyl_igr_mass_bifuel : Inport  Port=32  Interpolate=off
  Vxx_cyl_fill_mdl_ovlp_mass_bifuel : Inport  Port=33  Interpolate=off
  ASXX_MWIN_FLW_filupxxxxg_10ms : Subsystem  Tag=[RUNNABLE]  TreatAsAtomicUnit=on  RTWFileName=InAsiIaf_Filupxx_xxxxxg
      settings: AttributesFormatString=%<Tag>  RTWSystemCode=Nonreusable function  RTWFcnNameOpts=Use subsystem name  RTWFileNameOpts=User specified
  Vxx_cyl_fill_efy : Outport
  Vxx_cyl_fill_efy_fil : Outport  Port=2
  Vxx_cyl_fill_efy_intk_mfld_prs_atm_prs_cor : Outport  Port=3
  Vxx_cyl_fill_efy_sp : Outport  Port=4
  Vxx_cyl_fill_efy_fil_sp : Outport  Port=5
  Vxx_cyl_igr_mass : Outport  Port=6
  Vxx_eng_vol_fill_efy : Outport  Port=7
  Vxx_eng_vol_fill_efy_fil : Outport  Port=8
  Vxx_cyl_fill_trap_efy_opt : Outport  Port=9
  Vxx_cyl_fill_efy_dyn_cor : Outport  Port=10
  Vxx_cyl_fill_efy_temp_cor : Outport  Port=11
  wires:
  Vxx_cyl_fill_efy_vvt_intk_cor_fac_2_bifuel/1 -> ASXX_MWIN_FLW_filupxxxxg_10ms/20(Vxx_cyl_fill_efy_vvt_intk_cor_fac_2_bifuel)
  Vxx_intk_mfld_prs/1 -> ASXX_MWIN_FLW_filupxxxxg_10ms/2(Vxx_intk_mfld_prs)
  Vxx_cyl_fill_efy_bas_bifuel/1 -> ASXX_MWIN_FLW_filupxxxxg_10ms/6(Vxx_cyl_fill_efy_bas_bifuel)
  Vxx_cyl_fill_efy_vvt_intk_ex_cor/1 -> ASXX_MWIN_FLW_filupxxxxg_10ms/11(Vxx_cyl_fill_efy_vvt_intk_ex_cor)
  ASXX_MWIN_FLW_filupxxxxg_10ms/9(Vxx_cyl_fill_trap_efy_opt) -> Vxx_cyl_fill_trap_efy_opt/1
  Vxx_vvt_ex_angl/1 -> ASXX_MWIN_FLW_filupxxxxg_10ms/26(Vxx_vvt_ex_angl)
  Vxx_cyl_fill_efy_temp_cor_bifuel/1 -> ASXX_MWIN_FLW_filupxxxxg_10ms/7(Vxx_cyl_fill_efy_temp_cor_bifuel)
  Vxx_cyl_fill_efy_dyn_l_fill_fac_bifuel/1 -> ASXX_MWIN_FLW_filupxxxxg_10ms/16(Vxx_cyl_fill_efy_dyn_l_fill_fac_bifuel)
  ASXX_MWIN_FLW_filupxxxxg_10ms/3(Vxx_cyl_fill_efy_intk_mfld_prs_atm_prs_cor) -> Vxx_cyl_fill_efy_intk_mfld_prs_atm_prs_cor/1
  ASXX_MWIN_FLW_filupxxxxg_10ms/6(Vxx_cyl_igr_mass) -> Vxx_cyl_igr_mass/1
  ASXX_MWIN_FLW_filupxxxxg_10ms/4(Vxx_cyl_fill_efy_sp) -> Vxx_cyl_fill_efy_sp/1
  Vxx_tq_fuel_typ_rat/1 -> ASXX_MWIN_FLW_filupxxxxg_10ms/4(Vxx_tq_fuel_typ_rat)
  ASXX_MWIN_FLW_filupxxxxg_10ms/7(Vxx_eng_vol_fill_efy) -> Vxx_eng_vol_fill_efy/1
  Vxx_cyl_fill_efy_vvt_intk_cor_fac_1_bifuel/1 -> ASXX_MWIN_FLW_filupxxxxg_10ms/19(Vxx_cyl_fill_efy_vvt_intk_cor_fac_1_bifuel)
  Vnx_eng_1st_sta_stt/1 -> ASXX_MWIN_FLW_filupxxxxg_10ms/9(Vnx_eng_1st_sta_stt)
  Vxx_mdl_ref_ex_mfld_prs/1 -> ASXX_MWIN_FLW_filupxxxxg_10ms/30(Vxx_mdl_ref_ex_mfld_prs)
  ASXX_MWIN_FLW_filupxxxxg_10ms/5(Vxx_cyl_fill_efy_fil_sp) -> Vxx_cyl_fill_efy_fil_sp/1
  Vxx_eng_cool_temp/1 -> ASXX_MWIN_FLW_filupxxxxg_10ms/8(Vxx_eng_cool_temp)
  Vxx_vvl_intk_l_lift_rat/1 -> ASXX_MWIN_FLW_filupxxxxg_10ms/21(Vxx_vvl_intk_l_lift_rat)
  Vxx_avg_eng_spd/1 -> ASXX_MWIN_FLW_filupxxxxg_10ms/1(Vxx_avg_eng_spd)
  Vxx_vvt_intk_angl_cls/1 -> ASXX_MWIN_FLW_filupxxxxg_10ms/25(Vxx_vvt_intk_angl_cls)
  Vxx_vvt_intk_angl/1 -> ASXX_MWIN_FLW_filupxxxxg_10ms/3(Vxx_vvt_intk_angl)
  Vxx_cyl_fill_efy_dyn_cor_cool_temp_bifuel/1 -> ASXX_MWIN_FLW_filupxxxxg_10ms/17(Vxx_cyl_fill_efy_dyn_cor_cool_temp_bifuel)
  Vxx_cyl_fill_efy_dyn_cor_accel_t_cst_bifuel/1 -> ASXX_MWIN_FLW_filupxxxxg_10ms/13(Vxx_cyl_fill_efy_dyn_cor_accel_t_cst_bifuel)
  Vxx_cyl_fill_efy_dyn_cor_thrml_bifuel/1 -> ASXX_MWIN_FLW_filupxxxxg_10ms/14(Vxx_cyl_fill_efy_dyn_cor_thrml_bifuel)
  Vxx_vvl_intk_l_lift_rat_sp/1 -> ASXX_MWIN_FLW_filupxxxxg_10ms/22(Vxx_vvl_intk_l_lift_rat_sp)
  Vxx_cyl_fill_efy_dyn_cor_atm_prs_bifuel/1 -> ASXX_MWIN_FLW_filupxxxxg_10ms/15(Vxx_cyl_fill_efy_dyn_cor_atm_prs_bifuel)
  Vxx_cyl_fill_efy_dyn_cor_decl_t_cst_bifuel/1 -> ASXX_MWIN_FLW_filupxxxxg_10ms/18(Vxx_cyl_fill_efy_dyn_cor_decl_t_cst_bifuel)
  ASXX_MWIN_FLW_filupxxxxg_10ms/2(Vxx_cyl_fill_efy_fil) -> Vxx_cyl_fill_efy_fil/1
  Vxx_ex_mfld_prs/1 -> ASXX_MWIN_FLW_filupxxxxg_10ms/29(Vxx_ex_mfld_prs)
  Vxx_ex_mfld_temp/1 -> ASXX_MWIN_FLW_filupxxxxg_10ms/27(Vxx_ex_mfld_temp)
  ASXX_MWIN_FLW_filupxxxxg_10ms/8(Vxx_eng_vol_fill_efy_fil) -> Vxx_eng_vol_fill_efy_fil/1
  Vxx_intk_vlv_temp/1 -> ASXX_MWIN_FLW_filupxxxxg_10ms/5(Vxx_intk_vlv_temp)
  ASXX_MWIN_FLW_filupxxxxg_10ms/1(Vxx_cyl_fill_efy) -> Vxx_cyl_fill_efy/1
  Vxx_vvt_intk_angl_cls_l_lift/1 -> ASXX_MWIN_FLW_filupxxxxg_10ms/24(Vxx_vvt_intk_angl_cls_l_lift)
  Vbx_aj_accel_decl/1 -> ASXX_MWIN_FLW_filupxxxxg_10ms/12(Vbx_aj_accel_decl)
  Vxx_pft_rel_diff_prs/1 -> ASXX_MWIN_FLW_filupxxxxg_10ms/28(Vxx_pft_rel_diff_prs)
  Vxx_vvt_ex_angl_cls/1 -> ASXX_MWIN_FLW_filupxxxxg_10ms/23(Vxx_vvt_ex_angl_cls)
  Vxx_atm_prs/1 -> ASXX_MWIN_FLW_filupxxxxg_10ms/10(Vxx_atm_prs)
  Vxx_cyl_fill_mdl_pump_mass_bas_bifuel/1 -> ASXX_MWIN_FLW_filupxxxxg_10ms/31(Vxx_cyl_fill_mdl_pump_mass_bas_bifuel)
  Vxx_cyl_igr_mass_bifuel/1 -> ASXX_MWIN_FLW_filupxxxxg_10ms/32(Vxx_cyl_igr_mass_bifuel)
  Vxx_cyl_fill_mdl_ovlp_mass_bifuel/1 -> ASXX_MWIN_FLW_filupxxxxg_10ms/33(Vxx_cyl_fill_mdl_ovlp_mass_bifuel)
  ASXX_MWIN_FLW_filupxxxxg_10ms/10(Vxx_cyl_fill_mdl_intk_mfld_prs_diff_cor) -> Vxx_cyl_fill_efy_dyn_cor/1
  ASXX_MWIN_FLW_filupxxxxg_10ms/11(Vxx_cyl_fill_mdl_ex_mfld_prs_rat_cor) -> Vxx_cyl_fill_efy_temp_cor/1

== system Test_Model_HR12_2016/ASXX_MWIN_FLW_G/ASXX_MWIN_FLW_G/ASXX_MWIN_FLW_pumpflwxxg ==
  Vxx_cyl_fill_efy : Inport  Interpolate=off
  Vxx_min_intk_mfld_prs_pump_flow : Inport  Port=2  Interpolate=off
  Vxx_intk_mfld_prs : Inport  Port=3  Interpolate=off
  Vxx_intk_vlv_temp : Inport  Port=4  Interpolate=off
  Vxx_mgstr_gs_convs : Inport  Port=5  Interpolate=off
  ASXX_MWIN_FLW_pumpflwxxg_10ms : Subsystem  Tag=[RUNNABLE]  TreatAsAtomicUnit=on  RTWFileName=InAsiIaf_Airwhxx_xxxxxg
      settings: AttributesFormatString=%<Tag>  RTWSystemCode=Nonreusable function  RTWFcnNameOpts=Use subsystem name  RTWFileNameOpts=User specified
  Vxx_cyl_pump_flow : Outport
  wires:
  Vxx_mgstr_gs_convs/1 -> ASXX_MWIN_FLW_pumpflwxxg_10ms/5(Vxx_mgstr_gs_convs)
  Vxx_intk_vlv_temp/1 -> ASXX_MWIN_FLW_pumpflwxxg_10ms/4(Vxx_intk_vlv_temp)
  ASXX_MWIN_FLW_pumpflwxxg_10ms/1(Vxx_cyl_pump_flow) -> Vxx_cyl_pump_flow/1
  Vxx_cyl_fill_efy/1 -> ASXX_MWIN_FLW_pumpflwxxg_10ms/1(Vxx_cyl_fill_efy)
  Vxx_intk_mfld_prs/1 -> ASXX_MWIN_FLW_pumpflwxxg_10ms/3(Vxx_intk_mfld_prs)
  Vxx_min_intk_mfld_prs_pump_flow/1 -> ASXX_MWIN_FLW_pumpflwxxg_10ms/2(Vxx_min_intk_mfld_prs_pump_flow)

== system Test_Model_HR12_2016/ASXX_MWIN_FLW_G/ASXX_MWIN_FLW_G/ASXX_MWIN_FLW_pzeroxxxxg ==
  Vxx_avg_eng_spd : Inport  Interpolate=off
  Vxx_intk_mfld_prs : Inport  Port=2  Interpolate=off
  Vxx_atm_prs : Inport  Port=3  Interpolate=off
  Vxx_pft_rel_diff_prs : Inport  Port=4  Interpolate=off
  ASXX_MWIN_FLW_pzeroxxxxg_10ms : Subsystem  Tag=[RUNNABLE]  TreatAsAtomicUnit=on  RTWFileName=InAsiIaf_Pzeroxx_xxxxxg
      settings: AttributesFormatString=%<Tag>  RTWSystemCode=Nonreusable function  RTWFcnNameOpts=Use subsystem name  RTWFileNameOpts=User specified
  Vxx_min_map_maf : Outport
  Vxx_min_intk_mfld_prs_pump_flow : Outport  Port=2
  wires:
  ASXX_MWIN_FLW_pzeroxxxxg_10ms/2(Vxx_min_intk_mfld_prs_pump_flow) -> Vxx_min_intk_mfld_prs_pump_flow/1
  Vxx_avg_eng_spd/1 -> ASXX_MWIN_FLW_pzeroxxxxg_10ms/1(Vxx_avg_eng_spd)
  ASXX_MWIN_FLW_pzeroxxxxg_10ms/1(Vxx_min_map_maf) -> Vxx_min_map_maf/1
  Vxx_atm_prs/1 -> ASXX_MWIN_FLW_pzeroxxxxg_10ms/3(Vxx_atm_prs)
  Vxx_intk_mfld_prs/1 -> ASXX_MWIN_FLW_pzeroxxxxg_10ms/2(Vxx_intk_mfld_prs)
  Vxx_pft_rel_diff_prs/1 -> ASXX_MWIN_FLW_pzeroxxxxg_10ms/4(Vxx_pft_rel_diff_prs)

== system Test_Model_HR12_2016/ASXX_MWIN_FLW_G/ASXX_MWIN_FLW_G/ASXX_MWIN_FLW_trapexxxxg ==
  Vxx_avg_eng_spd : Inport  Interpolate=off
  Vxx_cyl_fill_efy_intk_mfld_prs_atm_prs_cor : Inport  Port=2  Interpolate=off
  Vxx_vvt_intk_angl : Inport  Port=3  Interpolate=off
  Vxx_vvt_ex_angl : Inport  Port=4  Interpolate=off
  ASXX_MWIN_FLW_trapexxxxg_10ms : Subsystem  Tag=[RUNNABLE]  TreatAsAtomicUnit=on  RTWFileName=InAsiIaf_Trapexx_xxxxxg
      settings: AttributesFormatString=%<Tag>  RTWSystemCode=Nonreusable function  RTWFcnNameOpts=Use subsystem name  RTWFileNameOpts=User specified
  Vxx_cyl_fill_trap_efy_vvt_intk_ex_cor : Outport
  wires:
  Vxx_avg_eng_spd/1 -> ASXX_MWIN_FLW_trapexxxxg_10ms/1(Vxx_avg_eng_spd)
  Vxx_vvt_intk_angl/1 -> ASXX_MWIN_FLW_trapexxxxg_10ms/3(Vxx_vvt_intk_angl)
  Vxx_cyl_fill_efy_intk_mfld_prs_atm_prs_cor/1 -> ASXX_MWIN_FLW_trapexxxxg_10ms/2(Vxx_cyl_fill_efy_intk_mfld_prs_atm_prs_cor)
  ASXX_MWIN_FLW_trapexxxxg_10ms/1(Vxx_cyl_fill_trap_efy_vvt_intk_ex_cor) -> Vxx_cyl_fill_trap_efy_vvt_intk_ex_cor/1
  Vxx_vvt_ex_angl/1 -> ASXX_MWIN_FLW_trapexxxxg_10ms/4(Vxx_vvt_ex_angl)

== system Test_Model_HR12_2016/ASXX_MWIN_FLW_G/ASXX_MWIN_FLW_G/ASXX_MWIN_FLW_trapinxxxg ==
  Vxx_avg_eng_spd : Inport  Interpolate=off
  Vxx_cyl_fill_efy_intk_mfld_prs_atm_prs_cor : Inport  Port=2  Interpolate=off
  Vxx_cyl_fill_trap_efy_vvt_intk_ex_cor : Inport  Port=3  Interpolate=off
  Vxx_cyl_fill_trap_efy_opt : Inport  Port=4  Interpolate=off
  ASXX_MWIN_FLW_trapinxxxg_10ms : Subsystem  Tag=[RUNNABLE]  TreatAsAtomicUnit=on  RTWFileName=InAsiIaf_Trapinx_xxxxxg
      settings: AttributesFormatString=%<Tag>  RTWSystemCode=Nonreusable function  RTWFcnNameOpts=Use subsystem name  RTWFileNameOpts=User specified
  Vxx_cyl_fill_trap_efy : Outport
  Vxx_eng_trap_fill_efy : Outport  Port=2
  wires:
  Vxx_cyl_fill_efy_intk_mfld_prs_atm_prs_cor/1 -> ASXX_MWIN_FLW_trapinxxxg_10ms/2(Vxx_cyl_fill_efy_intk_mfld_prs_atm_prs_cor)
  Vxx_cyl_fill_trap_efy_opt/1 -> ASXX_MWIN_FLW_trapinxxxg_10ms/4(Vxx_cyl_fill_trap_efy_opt)
  ASXX_MWIN_FLW_trapinxxxg_10ms/2(Vxx_eng_trap_fill_efy) -> Vxx_eng_trap_fill_efy/1
  Vxx_cyl_fill_trap_efy_vvt_intk_ex_cor/1 -> ASXX_MWIN_FLW_trapinxxxg_10ms/3(Vxx_cyl_fill_trap_efy_vvt_intk_ex_cor)
  Vxx_avg_eng_spd/1 -> ASXX_MWIN_FLW_trapinxxxg_10ms/1(Vxx_avg_eng_spd)
  ASXX_MWIN_FLW_trapinxxxg_10ms/1(Vxx_cyl_fill_trap_efy) -> Vxx_cyl_fill_trap_efy/1

== system Test_Model_HR12_2016/ASXX_MWIN_FLW_G/ASXX_MWIN_FLW_G/RTBSS_Vxx_cyl_fill_efy_intk_mfld_prs_atm_prs_cor ==
  Vxx_cyl_fill_efy_intk_mfld_prs_atm_prs_cor : Inport
  BusCreator : BusCreator  Inputs=2
  UnitDelay : UnitDelay  InitialCondition=double(single(101.3))  SampleTime=-1
      settings: AttributesFormatString=<initial=%<InitialCondition>>
  Vxx_cyl_fill_efy_intk_mfld_prs_atm_prs_cor_rt : Outport
  wires:
  BusCreator/1 -> Vxx_cyl_fill_efy_intk_mfld_prs_atm_prs_cor_rt/1
  UnitDelay/1 -> BusCreator/1  "Vxx_cyl_fill_efy_intk_mfld_prs_atm_prs_cor_pudt"
  Vxx_cyl_fill_efy_intk_mfld_prs_atm_prs_cor/1 -> BusCreator/2, UnitDelay/1  "Vxx_cyl_fill_efy_intk_mfld_prs_atm_prs_cor"

== system Test_Model_HR12_2016/ASXX_MWIN_TMP/ASXX_MWIN_TMP_ivlvtmd_20ms/B1_INTK_VLV_MIX_TEMP ==
  Vxx_thr_flow_20ms : Inport  Interpolate=off
  Vxx_intk_mfld_temp_20ms : Inport  Port=2  Interpolate=off
  Vxx_h_prs_egr_vlv_flow_20ms : Inport  Port=3  Interpolate=off
  Vxx_h_prs_egr_cool_ds_temp_20ms : Inport  Port=4  Interpolate=off
  AEMS_PROTECTED_DIVISION : AEMS_Standard_Library/MATH/AEMS_PROTECTED_DIVISION  Tag=[LIB]  out_mode=Default_Output -> Output  tolerance=0.0001
      settings: AttributesFormatString=%<MaskType>\nOutput when |Denominator| < Tolerance = %<out_mode>\nDenominator Tolerance = %<tolerance>
  Add1 : Sum  OutDataTypeStr=Inherit: Inherit via back propagation  InputSameDT=on
  Add9 : Sum  OutDataTypeStr=Inherit: Inherit via back propagation  InputSameDT=on
  Cxx_cp_spc_heat : Constant  Value=Cxx_thr_spc_heat
  Cxx_cp_spc_heat1 : Constant  Value=Cxx_egr_spc_heat
  Cxx_cp_spc_heat2 : Constant  Value=Cxx_thr_spc_heat
  Cxx_cp_spc_heat3 : Constant  Value=Cxx_egr_spc_heat
  DocBlock1 : simulink/Model-Wide Utilities/DocBlock  DocumentType=RTF
  Product{1..6} (6 alike) : Product  OutDataTypeStr=Inherit: Inherit via back propagation
  Saturation : Saturate  UpperLimit=250  LowerLimit=-50  RndMeth=Zero
      settings: AttributesFormatString=<limits=%<UpperLimit>/%<LowerLimit>>
  Saturation1 : Saturate  UpperLimit=215  LowerLimit=-40  RndMeth=Zero
      settings: AttributesFormatString=<limits=%<UpperLimit>/%<LowerLimit>>
  Saturation3 : Saturate  UpperLimit=200  LowerLimit=-40  RndMeth=Zero
      settings: AttributesFormatString=<limits=%<UpperLimit>/%<LowerLimit>>
  Vxx_mat_20ms : Outport
  Vxx_pid_0fh_a_20ms : Outport  Port=2
  Vxx_intk_vlv_mix_temp_20ms : Outport  Port=3
  wires:
  Product6/1 -> Add9/1
  Product5/1 -> Add9/2
  Product4/1 -> Add1/1
  Product3/1 -> Add1/2
  Vxx_h_prs_egr_vlv_flow_20ms/1 -> Product3/1, Product5/1
  Vxx_thr_flow_20ms/1 -> Product4/1, Product6/1
  Vxx_h_prs_egr_cool_ds_temp_20ms/1 -> Product1/2
  Cxx_cp_spc_heat/1 -> Product4/2
  Cxx_cp_spc_heat1/1 -> Product3/2
  Add9/1 -> AEMS_PROTECTED_DIVISION/1
  Add1/1 -> AEMS_PROTECTED_DIVISION/2
  Vxx_intk_mfld_temp_20ms/1 -> Product2/2, AEMS_PROTECTED_DIVISION/3
  Saturation/1 -> Vxx_intk_vlv_mix_temp_20ms/1  "Vxx_intk_vlv_mix_temp_20ms"
  Cxx_cp_spc_heat2/1 -> Product2/1
  Cxx_cp_spc_heat3/1 -> Product1/1
  Product1/1 -> Product5/2
  Product2/1 -> Product6/2
  AEMS_PROTECTED_DIVISION/1 -> Saturation3/1, Saturation1/1, Saturation/1
  Saturation3/1 -> Vxx_mat_20ms/1  "Vxx_mat_20ms"
  Saturation1/1 -> Vxx_pid_0fh_a_20ms/1  "Vxx_pid_0fh_a_20ms"

== system Test_Model_HR12_2016/ASXX_MWIN_TMP/ASXX_MWIN_TMP_ivlvtmd_20ms/B2_INTK_VLV_TEMP ==
  Vxx_intk_vlv_mix_temp_20ms : Inport  Interpolate=off
  Vxx_eng_cool_temp_20ms : Inport  Port=2  Interpolate=off
  Vxx_eng_cool_pump_flow_sp_20ms : Inport  Port=3  Interpolate=off
  Vxx_intk_vlv_flow_20ms : Inport  Port=4  Interpolate=off
  AEMS_LUT_2D : AEMS_Standard_Library/LOOKUP_TABLES/AEMS_LUT_2D  Tag=[LIB]  map_x=Cxb_eng_cool_pump_flow_intk_vlv_efy  map_y=Cxb_intk_vlv_flow_efy  carto=Cxm_eng_cool_pump_intk_vlv_flow_efy
      settings: AttributesFormatString=%<MaskType>\nBkPX=%<map_x>\nBkPY=%<map_y>\nMAP=%<carto>
  DocBlock1 : simulink/Model-Wide Utilities/DocBlock  DocumentType=RTF
  Embedded MATLAB Function2 : MATLAB Function  TreatAsAtomicUnit=on
  Product : Product  OutDataTypeStr=Inherit: Inherit via back propagation
  Saturation3 : Saturate  UpperLimit=200  LowerLimit=-50  RndMeth=Zero
      settings: AttributesFormatString=<limits=%<UpperLimit>/%<LowerLimit>>
  Scope6 : Scope  NumInputPorts=2
  Sum : Sum  OutDataTypeStr=Inherit: Inherit via back propagation  RndMeth=Zero  InputSameDT=on
  Sum1 : Sum  Inputs=-+  OutDataTypeStr=Inherit: Inherit via back propagation  RndMeth=Zero  InputSameDT=on
  Vxx_intk_vlv_temp_20ms : Outport
  wires:
  Product/1 -> Sum/2
  AEMS_LUT_2D/1 -> Product/2  "Vxx_eng_cool_pump_intk_vlv_flow_efy_20ms"
  Sum1/1 -> Product/1
  Sum/1 -> Scope6/1, Saturation3/1
  Vxx_eng_cool_temp_20ms/1 -> Embedded MATLAB Function2/2(Tco), Sum1/2
  Vxx_intk_vlv_mix_temp_20ms/1 -> Sum/1, Embedded MATLAB Function2/1(Tman), Sum1/1
  Saturation3/1 -> Vxx_intk_vlv_temp_20ms/1  "Vxx_intk_vlv_temp_20ms"
  Vxx_intk_vlv_flow_20ms/1 -> Embedded MATLAB Function2/3(QA), AEMS_LUT_2D/2
  Vxx_eng_cool_pump_flow_sp_20ms/1 -> AEMS_LUT_2D/1
  Embedded MATLAB Function2/1(Tvlv) -> Scope6/2  "Masp_est"

== system Test_Model_HR12_2016/ASXX_MWIN_FLW_G/ASXX_MWIN_FLW_G/ASXX_MWIN_FLW_filupexxxg/ASXX_MWIN_FLW_filupexxxg_10ms ==
  Vxx_avg_eng_spd : Inport  Interpolate=off
  Vxx_cyl_fill_efy_intk_mfld_prs_atm_prs_cor_pudt : Inport  Port=2  Interpolate=off
  Vxx_vvt_intk_angl : Inport  Port=3  Interpolate=off
  Vxx_vvt_ex_angl : Inport  Port=4  Interpolate=off
  Vxx_cyl_fill_efy_vvt_ex_cor_fac_1_bifuel : Inport  Port=5  Interpolate=off
  Vxx_cyl_fill_efy_vvt_ex_cor_fac_2_bifuel : Inport  Port=6  Interpolate=off
  Vxx_tq_fuel_typ_rat : Inport  Port=7  Interpolate=off
  Cbx_vvtc_in_angl_ofs : Constant  Value=Cbx_ex_vvt_conf
  DocBlock : Subsystem  mask(DocBlock){ECoderFlag=, DocumentType=Text}
      mask prompts: ECoderFlag "Simulink:blocks:docblockEmbeddedCoderFlagLabel"; DocumentType "Simulink:blocks:docblockDocTypeLabel"
      mask help: Use this block to save long descriptive text with the model. Double-clicking the block will open an editor.
      mask TypeOptions DocumentType: Text | RTF | HTML
      mask Display:
      | plot([.8 0 0 1 1 .8 .8 1],[1 1 0 0 .8 1 .8 .8]);
      | text(.5,.6,'DOC','horizontalalignment','center');
      | text(.95,.05,get_param(gcb,'DocumentType'),'verticalalignment','bottom','horizontalalignment','right');
  Filupexxxg : Subsystem  TreatAsAtomicUnit=on
  Vxx_cyl_fill_efy_vvt_intk_ex_cor : Outport  SourceOfInitialOutputValue=Input signal
  wires:
  Vxx_avg_eng_spd/1 -> Filupexxxg/1(Vxx_avg_eng_spd)  "Vxx_avg_eng_spd"
  Vxx_cyl_fill_efy_intk_mfld_prs_atm_prs_cor_pudt/1 -> Filupexxxg/2(Vxx_cyl_fill_efy_intk_mfld_prs_atm_prs_cor_pudt)  "Vxx_cyl_fill_efy_intk_mfld_prs_atm_prs_cor_pudt"
  Vxx_vvt_intk_angl/1 -> Filupexxxg/3(Vxx_vvt_intk_angl)  "Vxx_vvt_intk_angl"
  Vxx_vvt_ex_angl/1 -> Filupexxxg/4(Vxx_vvt_ex_angl)  "Vxx_vvt_ex_angl"
  Vxx_cyl_fill_efy_vvt_ex_cor_fac_1_bifuel/1 -> Filupexxxg/5(Vxx_cyl_fill_efy_vvt_ex_cor_fac_1_bifuel)  "Vxx_cyl_fill_efy_vvt_ex_cor_fac_1_bifuel"
  Vxx_cyl_fill_efy_vvt_ex_cor_fac_2_bifuel/1 -> Filupexxxg/6(Vxx_cyl_fill_efy_vvt_ex_cor_fac_2_bifuel)  "Vxx_cyl_fill_efy_vvt_ex_cor_fac_2_bifuel"
  Vxx_tq_fuel_typ_rat/1 -> Filupexxxg/7(Vxx_tq_fuel_typ_rat)  "Vxx_tq_fuel_typ_rat"
  Cbx_vvtc_in_angl_ofs/1 -> Filupexxxg/Enable
  Filupexxxg/1(Vxx_cyl_fill_efy_vvt_intk_ex_cor) -> Vxx_cyl_fill_efy_vvt_intk_ex_cor/1
